simulink model "solar_panel"  (R2021a)
settings: Solver=VariableStepAuto  StartTime=0.0  StopTime=24*60*60  RelTol=1e-3
undefined symbols (not defined in the file or in its folder): V2G
settings Model: Creator=emilm  LastModifiedBy=emilm

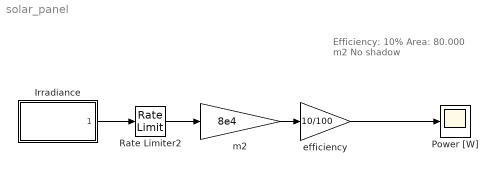
== system solar_panel ==
  note: Efficiency: 10%
      | Area: 80.000 m2
      | No shadow
  Irradiance : Subsystem
      mask init:
      | load power_V2G
      mask Display: plot(V2G.IRRADIANCE.time,V2G.IRRADIANCE.SUN)
  Power [W] : Scope
  Rate Limiter2 : RateLimiter  RisingSlewLimit=1e4  FallingSlewLimit=-1e4  SampleTimeMode=inherited
  efficiency : Gain  Gain=10/100
  m2 : Gain  Gain=8e4
  wires:
  Rate Limiter2/1 -> m2/1
  Irradiance/1(" ") -> Rate Limiter2/1
  m2/1 -> efficiency/1
  efficiency/1 -> Power [W]/1

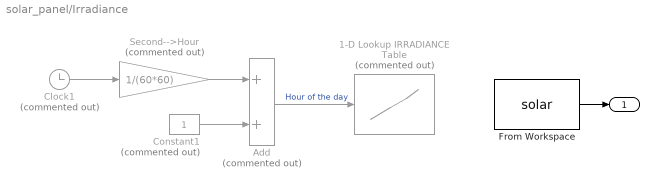
== system solar_panel/Irradiance ==
  1-D Lookup IRRADIANCE Table : Lookup_n-D  Commented=on  NumberOfTableDimensions=1  BreakpointsForDimension1=V2G.IRRADIANCE.time  BeginIndexSearchUsingPreviousIndexResult=on  Table=V2G.IRRADIANCE.SUN  InternalRulePriority=Speed  RndMeth=Simplest  InputSameDT=on
  Add : Sum  Commented=on
  Clock1 : Clock  Commented=on
  Constant1 : Constant  Commented=on
  From Workspace : FromWorkspace  VariableName=solar  SampleTime=24*60*60/1381  Interpolate=off  ZeroCross=off  OutputAfterFinalValue=Cyclic repetition
  Second-->Hour : Gain  Commented=on  Gain=1/(60*60)
  " " : Outport  VectorParamsAs1DForOutWhenUnconnected=off
  wires:
  Constant1/1 -> Add/2
  Add/1 -> 1-D Lookup IRRADIANCE Table/1  "Hour of the day"
  Clock1/1 -> Second-->Hour/1
  Second-->Hour/1 -> Add/1
  From Workspace/1 -> " "/1
